simulink model "spring_mass_model_01"  (R2014a)
settings: Solver=FixedStepDiscrete  StartTime=0.0  StopTime=inf  FixedStep=sample_time  RelTol=1e-3
values from neighbouring files (symbols this model uses):
  g = g_real    (= 9.803)    [max_motor_torques.m]
  l0_leg = 0.97    [max_motor_torques.m]
  l0_virtual = sqrt(d^2+l0_leg^2-2*d*l0_leg*cos(phi0))    [max_motor_torques.m]
undefined symbols (not defined in the file or in its folder): alpha_apex, alpha_max, alpha_min, boom_mount_angle, c_energy, contact_threshold, control_start_time, d_y_boom_com_offset, d_y_boom_hip_offset, d_y_com, d_y_mount_to_com, desired_torso_angle, DiscIntNeverNeededParam, dt_thrust, dx_avg_desired, extra_leg_damping, F_thrust, fcut_contact, ff_energy_l, ff_energy_r, g_reduced, h_boom, i_limit_lateral, i_robot, initial_com_height, initial_dt, initial_dx, j_leg, j_rotor, j_segments, k0_virtual, k_placement, k_sea, kd_flight, kd_lateral, kd_leg_angle, kd_motor, kd_raibert, kd_torso, ki_lateral, kp_flight_max, kp_flight_min, kp_lateral, kp_leg_angle, kp_motor, kp_raibert, kp_torso, l0_max_angle_error, l0_min_angle_error, l0_min_flight_time, l_boom, l_boom_projected, l_max, l_min, l_retract_escape, l_retract_swing, l_seg, lambda1, lambda2, lateral_offset ... (+33)
libraries: simulink x22, simulink_extras x2
(part 1 of 3)
settings Model: xpc_rtwmakecfg_data=_xpcethercatlib_  BufferReuse=off  Creator=wmartin  LastModifiedBy=wmartin
settings SolverCC: EnableConcurrentExecution=on
settings DataIOCC: MaxDataPoints=1000000000  SaveFormat=StructureWithTime
settings OptimizationCC: BlockReduction=off  OptimizeBlockIOStorage=off  BufferReuse=off  GlobalBufferReuse=off  ExpressionFolding=off  ExpressionDepthLimit=2147483647  LocalBlockOutputs=off  SimCompilerOptimization=On
settings DebuggingCC: AlgebraicLoopMsg=error  UnderspecifiedInitializationDetection=Classic  StateNameClashWarn=warning
settings HardwareCC: ProdIntDivRoundTo=Zero  ProdEndianess=LittleEndian  ProdHWDeviceType=Generic->32-bit x86 compatible
settings ModelReferenceCC: UpdateModelReferenceTargets=IfOutOfDate  EnableParallelModelReferenceBuilds=on  ParallelModelReferenceMATLABWorkerInit=Copy Base Workspace
settings RTWCC: SystemTargetFile=slrt.tlc  TemplateMakefile=slrt_default_tmf  Description=Simulink Real-Time  RTWVerbose=off  ProcessScript=slrt_make_rtw_hook  RTWCompilerOptimization=On
settings CodeAppCC: MaxIdLength=127
settings TargetCC: CodeReplacementLibrary=XPC_BLAS  ParMdlRefBuildCompliant=on  ConcurrentExecutionCompliant=on  MatFileLogging=on  EnableShiftOperators=on  MATLABClassNameForMDSCustomization=xpcAperiodicCustomization

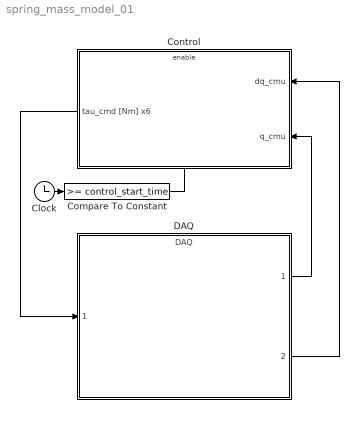
== system spring_mass_model_01 ==
  Clock : Clock
  Compare To Constant : simulink/Logic and Bit Operations/Compare To Constant  relop=>=  const=control_start_time  OutDataTypeStr=boolean
  Control : Subsystem
  DAQ : ModelReference  ModelNameDialog=DAQ  SimulationMode=Normal  ModelReferenceVersion=1.1655  CopyOfModelName=DAQ  DefaultDataLogging=on
  wires:
  DAQ/1 -> Control/2(q_cmu)
  DAQ/2 -> Control/1(dq_cmu)
  Clock/1 -> Compare To Constant/1
  Compare To Constant/1 -> Control/Enable
  Control/1(tau_cmd [Nm] x6) -> DAQ/1

== system spring_mass_model_01/Control ==
  dq_cmu : Inport
  q_cmu : Inport  Port=2
  Enable : EnablePort  StatesWhenEnabling=reset
  Actuator Control : ModelReference  ModelNameDialog=Actuator_Control  SimulationMode=Normal  ModelReferenceVersion=1.22  CopyOfModelName=Actuator_Control  DefaultDataLogging=on
  Behavior Control : Subsystem
  tau_cmd [Nm] x6 : Outport  InitialOutput=[0 0 0 0 0 0]
  wires:
  Behavior Control/1(Motor Torque Command [Nm] x6) -> Actuator Control/1
  dq_cmu/1 -> Behavior Control/1(dq_cmu), Actuator Control/4
  Actuator Control/1 -> tau_cmd [Nm] x6/1
  q_cmu/1 -> Behavior Control/2(q_cmu), Actuator Control/3
  Behavior Control/2(Force / Position Control [1/0] x4) -> Actuator Control/2

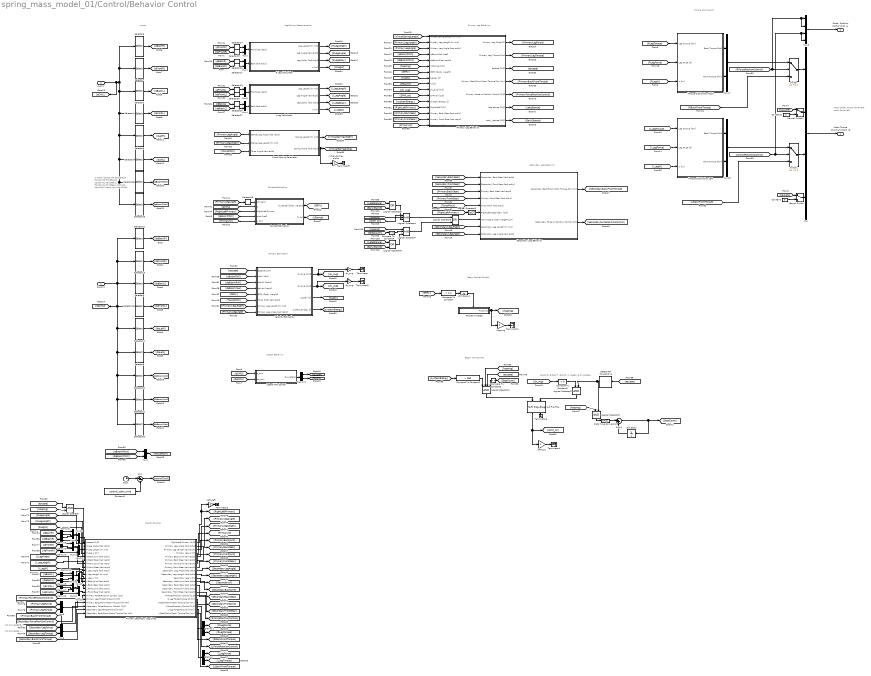
== system spring_mass_model_01/Control/Behavior Control ==
  note: not connected -->
  note: revert to raibert if velocity is negative on escape
  note: Motor Order:
      |
      | backR
      | frontR
      | latR
      | backL
      | frontL
      | latL
  note: q Order:
      |
      | backJointR
      | backGearR
      | frontJointR
      | frontGearR
      |
      | backJointL
      | backGearL
      | frontJointL
      | frontGearL
      |
      | latR
      | latL
      |
      | boomRoll
      | boomYaw
      | boomPitch
  note: Inputs
  note: Primary Leg Behavior
  note: Secondary Leg Behavior
  note: Torque Commands
  note: Lateral Behavior
  note: Leg/Spring Measurements
  note: Contact Estimation
  note: Velocity Estimation
  note: Begin SMM Control
  note: Begin Raibert Control
  note: Signal Routing
  note: not connected -->
  dq_cmu : Inport
  q_cmu : Inport  Port=2
  Clock : Clock
  Compare To Constant : simulink/Logic and Bit Operations/Compare To Constant  relop=>  const=1.4  OutDataTypeStr=boolean
  Compare To Constant1 : simulink/Logic and Bit Operations/Compare To Constant  relop=>  const=350  OutDataTypeStr=boolean
  Compare To Constant2 : simulink/Logic and Bit Operations/Compare To Constant  relop=<  const=0  OutDataTypeStr=boolean  ZeroCross=off
  Compare To Constant3 : simulink/Logic and Bit Operations/Compare To Constant  relop=>  const=4  OutDataTypeStr=boolean
  Compare To Constant4 : simulink/Logic and Bit Operations/Compare To Constant  relop=>  const=2  OutDataTypeStr=boolean
  Constant : Constant  Value=0
  Constant1 : Constant  Value=0
  Constant2 : Constant  Value=control_start_time
  Contact Estimation : Subsystem
  Data Type Conversion : DataTypeConversion  OutDataTypeStr=uint32
  Demux{,1..10} (11 alike) : Demux  Outputs=2
  Detect Fall Nonpositive : simulink/Logic and Bit Operations/Detect Fall Nonpositive  vinit=0  InputProcessing=Inherited  OutDataTypeStr=boolean
  L Leg Calculator : Subsystem
  Lateral PID Control : Subsystem
  Logical Operator : Logic  IconShape=distinctive  AllPortsSameDT=off  OutDataTypeStr=boolean
  Logical Operator1 : Logic  Inputs=4  IconShape=distinctive  AllPortsSameDT=off  OutDataTypeStr=boolean
  Logical Operator2 : Logic  IconShape=distinctive  AllPortsSameDT=off  OutDataTypeStr=boolean
  Logical Operator3 : Logic  Operator=NOT  AllPortsSameDT=off  OutDataTypeStr=boolean
  Logical Operator4 : Logic  Inputs=3  AllPortsSameDT=off  OutDataTypeStr=boolean
  Logical Operator5 : Logic  IconShape=distinctive  AllPortsSameDT=off  OutDataTypeStr=boolean
  Logical Operator6 : Logic  Operator=OR  AllPortsSameDT=off  OutDataTypeStr=boolean
  Logical Operator7 : Logic  Inputs=3  AllPortsSameDT=off  OutDataTypeStr=boolean
  Logical Operator8 : Logic  Operator=OR  AllPortsSameDT=off  OutDataTypeStr=boolean
  Logical Operator9 : Logic  Operator=OR  AllPortsSameDT=off  OutDataTypeStr=boolean
  Manual Switch : ManualSwitch
  Manual Switch1 : ManualSwitch
  Mux : Mux
  Mux{1..2,4..18} (17 alike) : Mux  Inputs=2
  Mux3 : Mux
  Primary Leg Behavior : Subsystem
  Primary Secondary Leg Swap : Subsystem
  R Leg Calculator : Subsystem
  Raibert Initiated : Subsystem
  S-R Flip-Flop : simulink_extras/Flip Flops/S-R Flip-Flop  initial_condition=0
  SMM_on : Gain
  Secondary Leg Behavior : Subsystem
  Selector1 : Selector  InputPortWidth=13  Indices=[10]
  Selector10 : Selector  InputPortWidth=13  Indices=[7 8]
  Selector11 : Selector  InputPortWidth=13  Indices=[9]
  Selector12 : Selector  InputPortWidth=13  Indices=[1 2]
  Selector13 : Selector  InputPortWidth=13  Indices=[3 4]
  Selector{14..17,19,24..27} (9 alike) : Selector  InputPortWidth=2  Indices=[1]
  Selector18 : Selector  InputPortWidth=13  Indices=[13]
  Selector2 : Selector  InputPortWidth=13  Indices=[5 6]
  Selector20 : Selector  InputPortWidth=13  Indices=[13]
  Selector21 : Selector  InputPortWidth=13  Indices=[11]
  Selector22 : Selector  InputPortWidth=13  Indices=[12]
  Selector23 : Selector  InputPortWidth=13  Indices=[11]
  Selector4 : Selector  InputPortWidth=13  Indices=[7 8]
  Selector5 : Selector  InputPortWidth=13  Indices=[9]
  Selector6 : Selector  InputPortWidth=13  Indices=[1 2]
  Selector7 : Selector  InputPortWidth=13  Indices=[3 4]
  Selector8 : Selector  InputPortWidth=13  Indices=[10]
  Selector9 : Selector  InputPortWidth=13  Indices=[5 6]
  Sum : Sum  Inputs=|+-
  Sum1 : Sum  Inputs=|++  OutMin=0
  Switch : Switch  Criteria=u2 ~= 0
  Switch1 : Switch  Criteria=u2 ~= 0
  Terminator{,1..6} (7 alike) : Terminator
  Torque Distribution Left : Subsystem
  Torque Distribution Right : Subsystem
  Unit Delay : UnitDelay  SampleTime=-1
  Unit Delay1 : UnitDelay  SampleTime=sample_time
  Velocity Estimation : Subsystem
  Virtual Spring Calculator : Subsystem
  dx_avg : Gain
  dy_avg : Gain
  hopping : Gain
  right_left : Gain
  virtual_spring_alpha : Gain
  Motor Torque Command [Nm] x6 : Outport  OutputWhenDisabled=reset  InitialOutput=[0 0 0 0 0 0]
  Force / Position Control [1/0] x4 : Outport  Port=2  OutputWhenDisabled=reset  InitialOutput=[0 0 0 0 0 0]
  wires:
  Lateral PID Control/1(tau_lateral) -> Demux2/1
  [dqCMU] -> Lateral PID Control/2(dq_cmu)
  [qCMU] -> Lateral PID Control/1(q_cmu)
  Sum/1 -> [controlClock]
  Selector4/1 -> [qFrontL]
  Selector2/1 -> [qBackL]
  Selector7/1 -> [qFrontR]
  Selector6/1 -> [qBackR]
  Selector1/1 -> [qLatL]
  Selector5/1 -> [qLatR]
  Constant2/1 -> Sum/2
  Clock/1 -> Sum/1
  Constant1/1 -> Manual Switch1/2
  Constant/1 -> Manual Switch/2
  Mux/1 -> Motor Torque Command [Nm] x6/1
  Selector8/1 -> [dqLatL]
  Selector11/1 -> [dqLatR]
  Selector12/1 -> [dqBackR]
  Selector13/1 -> [dqFrontR]
  Selector9/1 -> [dqBackL]
  Selector10/1 -> [dqFrontL]
  [qBackR] -> Selector16/1
  [dqBackR] -> Selector17/1
  [qFrontR] -> Selector14/1
  [dqFrontR] -> Selector15/1
  Mux2/1 -> R Leg Calculator/1(Front [rad rad/s])
  Mux1/1 -> R Leg Calculator/2(Back [rad rad/s])
  R Leg Calculator/1("Leg Length [m m/s] ") -> [RLegLength]
  R Leg Calculator/2(Leg Angle [rad rad/s]) -> [RLegAngle]
  R Leg Calculator/3(Leg Splay [rad rad/s]) -> [RLegSplay]
  Demux2/1 -> [tauLatR]
  Demux2/2 -> [tauLatL]
  [tauLatR] -> Manual Switch1/1
  [tauLatL] -> Manual Switch/1
  [RLegW] -> Torque Distribution Right/3(w [m])
  Selector14/1 -> Mux2/1
  Selector15/1 -> Mux2/2
  Selector17/1 -> Mux1/2
  Selector16/1 -> Mux1/1
  [PrimaryW] -> Contact Estimation/5(w [m])
  q_cmu/1 -> Selector6/1, Selector7/1, Selector2/1, Selector4/1, Selector5/1, Selector18/1, Selector23/1, Selector1/1, [qCMU]
  Selector18/1 -> [qBoomPitch]
  [qBoomPitch] -> Contact Estimation/4(pitch [rad])
  [PrimaryLegAngle] -> Selector19/1
  Selector19/1 -> Contact Estimation/1(phi [rad])
  Contact Estimation/1(F_vertical [body weight]) -> [GRFy]
  Selector20/1 -> [dqBoomPitch]
  [RLegForce] -> Torque Distribution Right/2(Leg Force [N])
  [RLegTorque] -> Torque Distribution Right/1(Leg Torque [Nm])
  Selector22/1 -> [dqBoomYaw]
  Contact Estimation/2(Ts [s]) -> [tStance]
  [GRFy] -> Compare To Constant/1
  Raibert Initiated/1(Hopping?) -> hopping/1, [hopping]
  dq_cmu/1 -> Selector20/1, Selector22/1, Selector21/1, Selector8/1, Selector11/1, Selector10/1, [dqCMU], Selector12/1, Selector13/1, Selector9/1
  Selector21/1 -> [dqBoomRoll]
  Selector23/1 -> [qBoomRoll]
  [qBackL] -> Selector26/1
  [dqBackL] -> Selector27/1
  [qFrontL] -> Selector24/1
  [dqFrontL] -> Selector25/1
  Mux5/1 -> L Leg Calculator/1(Front [rad rad/s])
  Mux4/1 -> L Leg Calculator/2(Back [rad rad/s])
  L Leg Calculator/1("Leg Length [m m/s] ") -> [LLegLength]
  L Leg Calculator/2(Leg Angle [rad rad/s]) -> [LLegAngle]
  L Leg Calculator/3(Leg Splay [rad rad/s]) -> [LLegSplay]
  Selector24/1 -> Mux5/1
  Selector25/1 -> Mux5/2
  Selector27/1 -> Mux4/2
  Selector26/1 -> Mux4/1
  R Leg Calculator/4(w [m]) -> [RLegW]
  L Leg Calculator/4(w [m]) -> [LLegW]
  Primary Leg Behavior/3(escape [1/0]) -> [escape]
  [PrimaryLegLength] -> Primary Leg Behavior/2(Primary Leg Length [m m/s])
  [hopping] -> Primary Leg Behavior/6(hopping [1/0])
  [GRFy] -> Primary Leg Behavior/7(GRFy [body weight])
  [qBoomPitch] -> Primary Leg Behavior/4(qBoomPitch [rad])
  [dqBoomPitch] -> Primary Leg Behavior/5(dqBoomPitch [rad/s])
  [PrimaryLegAngle] -> Primary Leg Behavior/3(Primary Leg Angle [rad rad/s])
  Primary Leg Behavior/1(Primary Leg Force [N]) -> [PrimaryLegForce]
  Primary Leg Behavior/2(Primary Leg Torque [Nm]) -> [PrimaryLegTorque]
  Velocity Estimation/1(dx_avg [m/s]) -> dx_avg/1, [dx_avg]
  [qBoomRoll] -> Velocity Estimation/2(qRoll [rad])
  [dqBoomYaw] -> Velocity Estimation/4(dqYaw [rad/s])
  dx_avg/1 -> Terminator/1
  hopping/1 -> Terminator1/1
  [LLegTorque] -> Torque Distribution Left/1(Leg Torque [Nm])
  [LLegForce] -> Torque Distribution Left/2(Leg Force [N])
  [LLegW] -> Torque Distribution Left/3(w [m])
  [qCMU] -> Contact Estimation/2(q)
  [RightLeftPrimary] -> Contact Estimation/3(Right/Left Primary)
  [PrimaryBackGear] -> Secondary Leg Behavior/3(Primary Back Gear [rad rad/s])
  [SecondaryLegAngle] -> Secondary Leg Behavior/9(Secondary Leg Angle [rad rad/s])
  [SecondaryLegLength] -> Secondary Leg Behavior/8(Secondary Leg Length [m m/s])
  right_left/1 -> Terminator2/1
  [hopping] -> Logical Operator/2
  Compare To Constant/1 -> Unit Delay1/1
  Velocity Estimation/2(dy_avg [m/s]) -> dy_avg/1, [dy_avg]
  [tApex] -> Primary Leg Behavior/8(t_apex [s])
  Velocity Estimation/3(t_apex [s]) -> [tApex]
  [GRFy] -> Velocity Estimation/5(GRFy [body weight])
  [PrimaryLegAngle] -> Velocity Estimation/8(Primary Leg Angle [rad rad/s])
  [PrimaryLegLength] -> Velocity Estimation/7(Primary Leg Length [m m/s])
  dy_avg/1 -> Terminator5/1
  [dqBoomRoll] -> Velocity Estimation/3(dqRoll [rad/s])
  [dx_avg] -> Primary Leg Behavior/10(dx_avg [m/s])
  [tStance] -> Primary Leg Behavior/9(Ts [s])
  Velocity Estimation/4(system_energy [J]) -> [systemEnergy]
  [systemEnergy] -> Compare To Constant1/1
  S-R Flip-Flop/1 -> [SMM_on], SMM_on/1
  SMM_on/1 -> Terminator4/1
  Compare To Constant1/1 -> Logical Operator1/1
  [SMM_on] -> Primary Leg Behavior/11(SMM On [1/0])
  [systemEnergy] -> Primary Leg Behavior/12(System Energy [J])
  Logical Operator1/1 -> S-R Flip-Flop/1
  [escape] -> Logical Operator1/3
  [RightLeftPrimary] -> Primary Leg Behavior/13(Right/Left [1/0])
  [PrimaryLegAngle] -> Virtual Spring Calculator/1("Stance Leg Angle [rad rad/s] ")
  [PrimaryLegLength] -> Virtual Spring Calculator/2(Stance Leg Length [m m/s])
  Virtual Spring Calculator/1(Spring Length [m m/s]) -> [VirtualSpringLength]
  [TorsoPitch] -> Virtual Spring Calculator/3(Torso Angle [rad rad/s])
  Virtual Spring Calculator/2(Spring Alpha [rad rad/s]) -> virtual_spring_alpha/1, [VirtualSpringAlpha]
  [qBoomPitch] -> Mux7/1
  [dqBoomPitch] -> Mux7/2
  Mux7/1 -> [TorsoPitch]
  [TorsoPitch] -> Secondary Leg Behavior/5(Torso Pitch [rad rad/s])
  [TorsoPitch] -> Velocity Estimation/6(Torso Pitch [rad rad/s])
  [VirtualSpringLength] -> Primary Leg Behavior/1(Virtual Spring Length [m m/s])
  virtual_spring_alpha/1 -> Terminator3/1
  [dx_avg] -> Compare To Constant2/1
  Detect Fall Nonpositive/1 -> Logical Operator2/2, Logical Operator5/2
  Compare To Constant2/1 -> Logical Operator2/1
  Logical Operator2/1 -> S-R Flip-Flop/2
  S-R Flip-Flop/2 -> Terminator6/1
  Mux3/1 -> Force / Position Control [1/0] x4/1
  Primary Secondary Leg Swap/2(Primary Leg Angle [rad rad/s]) -> [PrimaryLegAngle]
  Primary Secondary Leg Swap/4(Primary Leg w [m]) -> [PrimaryW]
  Primary Secondary Leg Swap/3(Primary Leg Length [rad rad/s]) -> [PrimaryLegLength]
  [RLegAngle] -> Primary Secondary Leg Swap/2(R Leg Angle [rad rad/s])
  [RLegLength] -> Primary Secondary Leg Swap/3(R Leg Length [m m/s])
  [RLegW] -> Primary Secondary Leg Swap/4(R Leg w [m])
  [LLegAngle] -> Primary Secondary Leg Swap/9(L Leg Angle [rad rad/s])
  [LLegLength] -> Primary Secondary Leg Swap/10(L Leg Length [m m/s])
  [LLegW] -> Primary Secondary Leg Swap/11(L Leg w [m])
  [SecondaryLegForce] -> Mux6/1
  [SecondaryLegTorque] -> Mux6/2
  Mux6/1 -> Primary Secondary Leg Swap/20(Secondary Leg Force/Torque [N Nm])
  Mux8/1 -> Primary Secondary Leg Swap/17(Primary Leg Force/Torque [N Nm])
  [PrimaryLegTorque] -> Mux8/2
  [PrimaryLegForce] -> Mux8/1
  Primary Secondary Leg Swap/10(Secondary Leg Length [rad rad/s]) -> [SecondaryLegLength]
  Primary Secondary Leg Swap/9(Secondary Leg Angle [rad rad/s]) -> [SecondaryLegAngle]
  Primary Secondary Leg Swap/20(L Leg Force/Torque [N Nm]) -> Demux/1
  Demux/1 -> [LLegForce]
  Demux/2 -> [LLegTorque]
  Primary Secondary Leg Swap/17(R Leg Force/Torque [N Nm]) -> Demux1/1
  Demux1/1 -> [RLegForce]
  Demux1/2 -> [RLegTorque]
  [qFrontR] -> Demux3/1
  [dqFrontR] -> Demux4/1
  Mux9/1 -> Primary Secondary Leg Swap/5(R Back Joint [rad rad/s])
  Mux10/1 -> Primary Secondary Leg Swap/6(R Back Gear [rad rad/s])
  Mux11/1 -> Primary Secondary Leg Swap/7(R Front Joint [rad rad/s])
  Mux12/1 -> Primary Secondary Leg Swap/8(R Front Gear [rad rad/s])
  Demux3/1 -> Mux11/1
  Demux3/2 -> Mux12/1
  Demux4/1 -> Mux11/2
  Demux4/2 -> Mux12/2
  [dqBackR] -> Demux5/1
  [qBackR] -> Demux6/1
  Demux6/1 -> Mux9/1
  Demux6/2 -> Mux10/1
  Demux5/1 -> Mux9/2
  Demux5/2 -> Mux10/2
  [qFrontL] -> Demux7/1
  [dqFrontL] -> Demux8/1
  Mux16/1 -> Primary Secondary Leg Swap/12(L Back Joint [rad rad/s])
  Mux13/1 -> Primary Secondary Leg Swap/13(L Back Gear [rad rad/s])
  Mux14/1 -> Primary Secondary Leg Swap/14(L Front Joint [rad rad/s])
  Mux15/1 -> Primary Secondary Leg Swap/15(L Front Gear [rad rad/s])
  Demux7/1 -> Mux14/1
  Demux7/2 -> Mux15/1
  Demux8/1 -> Mux14/2
  Demux8/2 -> Mux15/2
  [dqBackL] -> Demux9/1
  [qBackL] -> Demux10/1
  Demux10/1 -> Mux16/1
  Demux10/2 -> Mux13/1
  Demux9/1 -> Mux16/2
  Demux9/2 -> Mux13/2
  [PrimaryForcePositionControl] -> Primary Secondary Leg Swap/16(Primary Force/Position Control [1/0])
  [SecondaryForcePositionControl] -> Primary Secondary Leg Swap/19(Secondary Force/Position Control [1/0])
  [PrimaryBackFrontTorque] -> Primary Secondary Leg Swap/18(Primary Back/Front Motor Torque [Nm Nm])
  [SecondaryBackFrontTorque] -> Primary Secondary Leg Swap/21(Secondary Back/Front Motor Torque [Nm Nm])
  Primary Secondary Leg Swap/5(Primary Back Joint [rad rad/s]) -> [PrimaryBackJoint]
  Primary Secondary Leg Swap/6(Primary Back Gear [rad rad/s]) -> [PrimaryBackGear]
  Primary Secondary Leg Swap/7(Primary Front Joint [rad rad/s]) -> [PrimaryFrontJoint]
  Primary Secondary Leg Swap/8(Primary Front Gear [rad rad/s]) -> [PrimaryFrontGear]
  Primary Secondary Leg Swap/12(Secondary Back Joint [rad rad/s]) -> [SecondaryBackJoint]
  Primary Secondary Leg Swap/13(Secondary Back Gear [rad rad/s]) -> [SecondaryBackGear]
  Primary Secondary Leg Swap/14(Secondary Front Joint [rad rad/s]) -> [SecondaryFrontJoint]
  Primary Secondary Leg Swap/15(Secondary Front Gear [rad rad/s]) -> [SecondaryFrontGear]
  Primary Secondary Leg Swap/11(Secondary Leg w [m]) -> [SecondaryW]
  Primary Secondary Leg Swap/19(L Force/Position Control [1/0]) -> [LForcePositionControl]
  Primary Secondary Leg Swap/16(R Force/Position Control [1/0]) -> [RForcePositionControl]
  Primary Secondary Leg Swap/18(R Back/Front Motor Torque [Nm Nm]) -> [RBackFrontTorque]
  Primary Secondary Leg Swap/21(L Back/Front Motor Torque [Nm Nm]) -> [LBackFrontTorque]
  Logical Operator/1 -> Primary Secondary Leg Swap/1(escape [1/0])
  Primary Secondary Leg Swap/1(Right/Left Primary [1/0]) -> right_left/1, [RightLeftPrimary]
  [escape] -> Velocity Estimation/1(escape [1/0])
  [PrimaryBackGear] -> Primary Leg Behavior/14(Primary Back Gear [rad rad/s])
  [PrimaryFrontGear] -> Primary Leg Behavior/15(Primary Front Gear [rad rad/s])
  Primary Leg Behavior/4(Primary Back/Front Motor Torque [Nm Nm]) -> [PrimaryBackFrontTorque]
  Primary Leg Behavior/5(Primary Force or Position Control [1/0]) -> [PrimaryForcePositionControl]
  [PrimaryFrontGear] -> Secondary Leg Behavior/4(Primary Front Gear [rad rad/s])
  [RightLeftPrimary] -> Logical Operator3/1
  Logical Operator3/1 -> Secondary Leg Behavior/6(Right/Left Secondary [1/0])
  [SecondaryFrontGear] -> Secondary Leg Behavior/2(Secondary Front Gear [rad rad/s])
  [SecondaryBackGear] -> Secondary Leg Behavior/1(Secondary Back Gear [rad rad/s])
  Secondary Leg Behavior/2(Secondary Force or Position Control [1/0]) -> [SecondaryForcePositionControl]
  Secondary Leg Behavior/1(Secondary Back/Front Motor Torque [Nm Nm]) -> [SecondaryBackFrontTorque]
  Primary Leg Behavior/6(late stance [1/0]) -> [LateStance]
  [RForcePositionControl] -> Mux3/2, Mux3/1, Switch/2
  [LForcePositionControl] -> Mux3/4, Mux3/3, Switch1/2
  Switch/1 -> Mux/1
  Manual Switch1/1 -> Mux/2
  Manual Switch/1 -> Mux/4
  Torque Distribution Right/2(Front Torque [Nm]) -> Mux17/2
  Torque Distribution Right/1(Back Torque [Nm]) -> Mux17/1
  Torque Distribution Left/1(Back Torque [Nm]) -> Mux18/1
  Torque Distribution Left/2(Front Torque [Nm]) -> Mux18/2
  Mux17/1 -> Switch/1
  [RBackFrontTorque] -> Switch/3
  Mux18/1 -> Switch1/1
  [LBackFrontTorque] -> Switch1/3
  Switch1/1 -> Mux/3
  [PrimaryW] -> Primary Leg Behavior/16(Primary w [m])
  Logical Operator4/1 -> Logical Operator6/1
  [escape] -> Detect Fall Nonpositive/1
  [hopping] -> Logical Operator1/2
  Unit Delay/1 -> Sum1/2
  Sum1/1 -> [StepCount], Unit Delay/1
  Logical Operator5/1 -> Data Type Conversion/1
  Data Type Conversion/1 -> Sum1/1
  [hopping] -> Logical Operator5/1
  [StepCount] -> Compare To Constant3/1
  Compare To Constant3/1 -> Logical Operator1/4
  [StepCount] -> Compare To Constant4/1
  [hopping] -> Logical Operator7/1
  Compare To Constant4/1 -> Logical Operator7/2
  Logical Operator7/1 -> Logical Operator6/2
  Logical Operator6/1 -> Secondary Leg Behavior/7(Move Leg to Apex Target [1/0])
  Primary Leg Behavior/7(early_stance [1/0]) -> [EarlyStance]
  [EarlyStance] -> Logical Operator8/2
  [LateStance] -> Logical Operator8/1
  [EarlyStance] -> Logical Operator9/2
  [LateStance] -> Logical Operator9/1
  [hopping] -> Logical Operator4/1
  [SMM_on] -> Logical Operator4/2
  Logical Operator8/1 -> Logical Operator4/3
  Logical Operator9/1 -> Logical Operator7/3
  [escape] -> Logical Operator/1
  Unit Delay1/1 -> Raibert Initiated/Enable

== system spring_mass_model_01/Control/Behavior Control/Contact Estimation ==
  phi [rad] : Inport
  q : Inport  Port=2
  Right/Left Primary : Inport  Port=3
  pitch [rad] : Inport  Port=4
  w [m] : Inport  Port=5
  Compare To Constant : simulink/Logic and Bit Operations/Compare To Constant  relop=>=  const=loaded_threshold  OutDataTypeStr=boolean
  Compare To Constant1 : simulink/Logic and Bit Operations/Compare To Constant  relop=>=  const=0.040  OutDataTypeStr=boolean
  Constant : Constant  Value=m_total_real*g
  Contact Time : Subsystem
  Detect Decrease : simulink/Logic and Bit Operations/Detect Decrease  vinit=0.0  InputProcessing=Inherited  OutDataTypeStr=boolean
  Divide : Product  Inputs=*/
  Divide1 : Product  Inputs=*/
  Gain3 : Gain  Gain=-1
  Last Contact Time : Subsystem
  Leg Torque Measurements : Subsystem
  Logical Operator : Logic  AllPortsSameDT=off  OutDataTypeStr=boolean
  Sum1 : Sum  Inputs=|+-
  Vertical Spring Force : Subsystem
  two_pole_filter : DiscreteTransferFcn  Numerator=[(1-2*exp(-fcut_contact*sample_time)+exp(-2*fcut_contact*sample_time)) 0 0]  Denominator=[1 (-2*exp(-fcut_contact*sample_time)) (exp(-2*fcut_contact*sample_time))]  SampleTime=sample_time
  F_vertical [body weight] : Outport
  Ts [s] : Outport  Port=2
  wires:
  Vertical Spring Force/1(Vertical Force [N]) -> two_pole_filter/1
  Constant/1 -> Divide/2
  two_pole_filter/1 -> Divide/1
  q/1 -> Leg Torque Measurements/1(q)
  Leg Torque Measurements/1(Back [Nm]) -> Sum1/1
  Leg Torque Measurements/2(Front [Nm]) -> Sum1/2
  Sum1/1 -> Divide1/1
  Divide1/1 -> Vertical Spring Force/3(Force [N])
  pitch [rad]/1 -> Vertical Spring Force/1(theta [rad])
  w [m]/1 -> Gain3/1
  Gain3/1 -> Divide1/2
  phi [rad]/1 -> Vertical Spring Force/2(phi [rad])
  Last Contact Time/1(Ts [s]) -> Ts [s]/1
  Contact Time/1(ts [s]) -> Last Contact Time/1(ts [s]), Compare To Constant1/1
  Compare To Constant/1 -> Detect Decrease/1, Contact Time/Enable
  Logical Operator/1 -> Last Contact Time/Trigger
  Detect Decrease/1 -> Logical Operator/1
  Compare To Constant1/1 -> Logical Operator/2
  Right/Left Primary/1 -> Leg Torque Measurements/2(Right/Left Stance [1/0])
  Divide/1 -> F_vertical [body weight]/1, Compare To Constant/1

== system spring_mass_model_01/Control/Behavior Control/L Leg Calculator ==
  Front [rad rad/s] : Inport
  Back [rad rad/s] : Inport  Port=2
  Demux1 : Demux  Outputs=2
  Gain1 : Gain  Gain=2*l_seg
  Gain2 : Gain  Gain=l_seg
  Gain3 : Gain  Gain=-1
  Gain4 : Gain  Gain=0.5
  Gain5 : Gain  Gain=0.5
  Gain6 : Gain  Gain=2
  Mux1 : Mux  Inputs=2
  Product : Product  RndMeth=Zero
  Sum4 : Sum  Inputs=+|+
  Sum5 : Sum  Inputs=+|-
  Trigonometric Function : Trigonometry  Operator=cos
  Trigonometric Function1 : Trigonometry
  "Leg Length [m m/s] " : Outport
  Leg Angle [rad rad/s] : Outport  Port=2
  Leg Splay [rad rad/s] : Outport  Port=3
  w [m] : Outport  Port=4
  wires:
  Gain5/1 -> Leg Angle [rad rad/s]/1
  Sum4/1 -> Gain5/1
  Mux1/1 -> "Leg Length [m m/s] "/1
  Sum5/1 -> Demux1/1, Leg Splay [rad rad/s]/1
  Gain2/1 -> Gain6/1, Product/1
  Demux1/1 -> Gain4/1
  Gain3/1 -> Product/2
  Demux1/2 -> Gain3/1
  Back [rad rad/s]/1 -> Sum5/1, Sum4/1
  Front [rad rad/s]/1 -> Sum4/2, Sum5/2
  Product/1 -> Mux1/2
  Trigonometric Function1/1 -> Gain2/1
  Gain1/1 -> Mux1/1
  Trigonometric Function/1 -> Gain1/1
  Gain4/1 -> Trigonometric Function/1, Trigonometric Function1/1
  Gain6/1 -> w [m]/1

== system spring_mass_model_01/Control/Behavior Control/Lateral PID Control ==
  note: FB Linearization
  q_cmu : Inport
  dq_cmu : Inport  Port=2
  -mgd : Gain  Gain=m_leg_motor*g*lateral_offset
  90deg : Constant  Value=pi/2
  Gain : Gain  Gain=-1
  Lateral Hip PID : Subsystem
  Motor Saturation : Saturate  UpperLimit=max_torque_lateral  LowerLimit=-max_torque_lateral
      settings: AttributesFormatString=Top: %<UpperLimit>\nBottom: %<LowerLimit>
  Mux : Mux  Inputs=2
  Sum1 : Sum  Inputs=|+-
  Sum2 : Sum  Inputs=-+|
  Sum3 : Sum  Inputs=++|
  Sum4 : Sum  Inputs=++|
  desired_velocity : Constant  Value=0
  lateral_sine : Gain  Commented=on  Gain=pi/180
  lateral_wave : Sin  Commented=on  Amplitude=5  Frequency=2*pi*(1/2)  SampleTime=0
  select_dqLateral : Selector  InputPortWidth=13  Indices=[9 10]
  select_qLateral : Selector  InputPortWidth=13  Indices=[9 10]
  sin : Trigonometry
  spherical_correction_angle : Subsystem
  tau_lateral : Outport
  wires:
  lateral_wave/1 -> lateral_sine/1
  Lateral Hip PID/1(out) -> Sum4/2
  Sum2/1 -> Lateral Hip PID/1(position_error)
  q_cmu/1 -> spherical_correction_angle/1(q_cmu), select_qLateral/1
  select_dqLateral/1 -> Sum1/2
  dq_cmu/1 -> select_dqLateral/1
  Sum4/1 -> Motor Saturation/1
  desired_velocity/1 -> Sum1/1
  Sum1/1 -> Lateral Hip PID/2(velocity_error)
  Gain/1 -> Mux/2
  Mux/1 -> Sum2/2
  select_qLateral/1 -> Sum3/2, Sum2/1  "qLateral"
  Motor Saturation/1 -> tau_lateral/1
  spherical_correction_angle/1(lateral_correction [rad]) -> Mux/1, Gain/1
  -mgd/1 -> Sum4/1
  Sum3/1 -> sin/1
  90deg/1 -> Sum3/1
  sin/1 -> -mgd/1

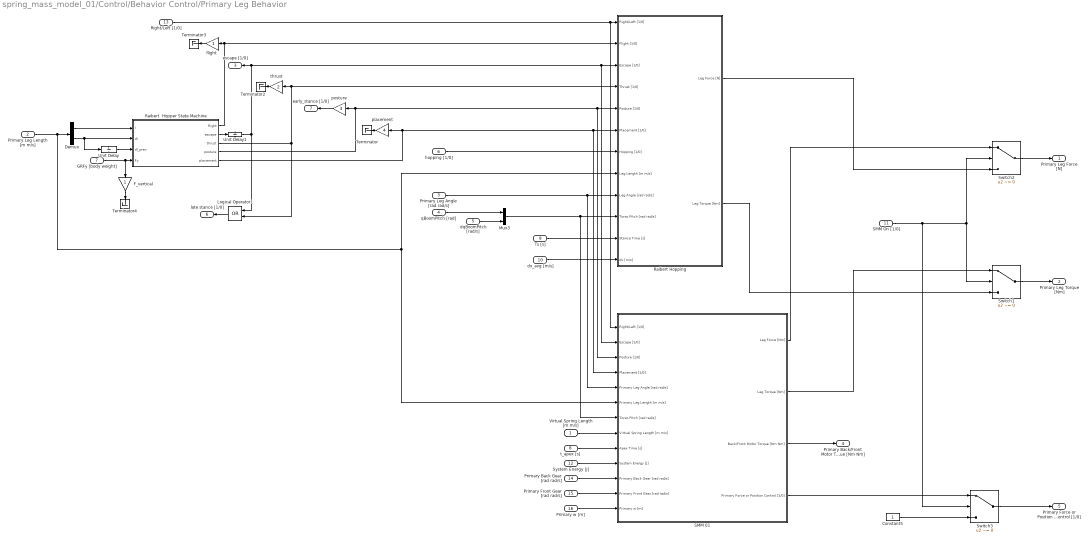
== system spring_mass_model_01/Control/Behavior Control/Primary Leg Behavior ==
  Virtual Spring Length [m m/s] : Inport
  Primary Leg Length [m m/s] : Inport  Port=2
  Primary Leg Angle [rad rad/s] : Inport  Port=3
  qBoomPitch [rad] : Inport  Port=4
  dqBoomPitch [rad/s] : Inport  Port=5
  hopping [1/0] : Inport  Port=6
  GRFy [body weight] : Inport  Port=7
  t_apex [s] : Inport  Port=8
  Ts [s] : Inport  Port=9
  dx_avg [m/s] : Inport  Port=10
  SMM On [1/0] : Inport  Port=11
  System Energy [J] : Inport  Port=12
  Right/Left [1/0] : Inport  Port=13
  Primary Back Gear [rad rad/s] : Inport  Port=14
  Primary Front Gear [rad rad/s] : Inport  Port=15
  Primary w [m] : Inport  Port=16
  Constant5 : Constant  OutDataTypeStr=boolean
  Demux : Demux  Outputs=2
  F_vertical : Gain
  Logical Operator1 : Logic  Operator=OR  AllPortsSameDT=off  OutDataTypeStr=boolean
  Mux3 : Mux  Inputs=2
  Raibert  Hopper State Machine : State Transition Table  TreatAsAtomicUnit=on
  Raibert Hopping : Subsystem
  SMM 01 : Subsystem
  Switch1 : Switch  Criteria=u2 ~= 0
  Switch2 : Switch  Criteria=u2 ~= 0
  Switch3 : Switch  Criteria=u2 ~= 0
  Terminator{,2..4} (4 alike) : Terminator
  Unit Delay : UnitDelay  SampleTime=-1
  Unit Delay1 : UnitDelay  SampleTime=sample_time
  flight : Gain
  placement : Gain  Gain=4
  posture : Gain  Gain=3
  thrust : Gain  Gain=2
  Primary Leg Force [N] : Outport
  Primary Leg Torque [Nm] : Outport  Port=2
  escape [1/0] : Outport  Port=3
  Primary Back/Front Motor Torque [Nm Nm] : Outport  Port=4
  Primary Force or Position Control [1/0] : Outport  Port=5
  late stance [1/0] : Outport  Port=6
  early_stance [1/0] : Outport  Port=7
  wires:
  Raibert  Hopper State Machine/4(posture) -> posture/1, SMM 01/3(Posture [1/0]), Raibert Hopping/5(Posture [1/0])
  Mux3/1 -> SMM 01/7(Torso Pitch [rad rad/s]), Raibert Hopping/10(Torso Pitch [rad rad/s])
  qBoomPitch [rad]/1 -> Mux3/1
  dqBoomPitch [rad/s]/1 -> Mux3/2
  Unit Delay/1 -> Raibert  Hopper State Machine/3(dl_prev)
  GRFy [body weight]/1 -> F_vertical/1, Raibert  Hopper State Machine/4(Fy)
  Demux/2 -> Unit Delay/1, Raibert  Hopper State Machine/2(dl)
  Raibert  Hopper State Machine/3(thrust) -> Logical Operator1/2, Raibert Hopping/4(Thrust [1/0]), thrust/1
  Raibert  Hopper State Machine/1(flight) -> flight/1, Raibert Hopping/2(Flight [1/0])
  Raibert  Hopper State Machine/5(placement) -> Raibert Hopping/6(Placement [1/0]), SMM 01/4(Placement [1/0]), placement/1
  placement/1 -> Terminator/1
  posture/1 -> early_stance [1/0]/1
  thrust/1 -> Terminator2/1
  Primary Leg Length [m m/s]/1 -> SMM 01/6(Primary Leg Length [m m/s]), Raibert Hopping/8(Leg Length [m m/s]), Demux/1
  F_vertical/1 -> Terminator4/1
  flight/1 -> Terminator3/1
  Demux/1 -> Raibert  Hopper State Machine/1(l)
  hopping [1/0]/1 -> Raibert Hopping/7(Hopping [1/0])
  SMM On [1/0]/1 -> Switch3/2, Switch1/2, Switch2/2
  Ts [s]/1 -> Raibert Hopping/11(Stance Time [s])
  dx_avg [m/s]/1 -> Raibert Hopping/12(dx [m/s])
  Raibert Hopping/1(Leg Force [N]) -> Switch2/3
  Raibert Hopping/2(Leg Torque [Nm]) -> Switch1/3
  Switch2/1 -> Primary Leg Force [N]/1
  Switch1/1 -> Primary Leg Torque [Nm]/1
  t_apex [s]/1 -> SMM 01/9(Apex Time [s])
  System Energy [J]/1 -> SMM 01/10(System Energy [J])
  SMM 01/1(Leg Force [Nm]) -> Switch2/1
  SMM 01/2(Leg Torque [Nm]) -> Switch1/1
  Right/Left [1/0]/1 -> SMM 01/1(Right/Left [1/0]), Raibert Hopping/1(Right/Left [1/0])
  Virtual Spring Length [m m/s]/1 -> SMM 01/8(Virtual Spring Length [m m/s])
  Primary Front Gear [rad rad/s]/1 -> SMM 01/12(Primary Front Gear [rad rad/s])
  Primary Back Gear [rad rad/s]/1 -> SMM 01/11(Primary Back Gear [rad rad/s])
  Primary Leg Angle [rad rad/s]/1 -> SMM 01/5(Primary Leg Angle [rad rad/s]), Raibert Hopping/9(Leg Angle [rad rad/s])
  SMM 01/3(Back/Front Motor Torque [Nm Nm]) -> Primary Back/Front Motor Torque [Nm Nm]/1
  Logical Operator1/1 -> late stance [1/0]/1
  Switch3/1 -> Primary Force or Position Control [1/0]/1
  Constant5/1 -> Switch3/3
  SMM 01/4(Primary Force or Position Control [1/0]) -> Switch3/1
  Primary w [m]/1 -> SMM 01/13(Primary w [m])
  Raibert  Hopper State Machine/2(escape) -> Unit Delay1/1
  Unit Delay1/1 -> SMM 01/2(Escape [1/0]), Raibert Hopping/3(Escape [1/0]), escape [1/0]/1, Logical Operator1/1

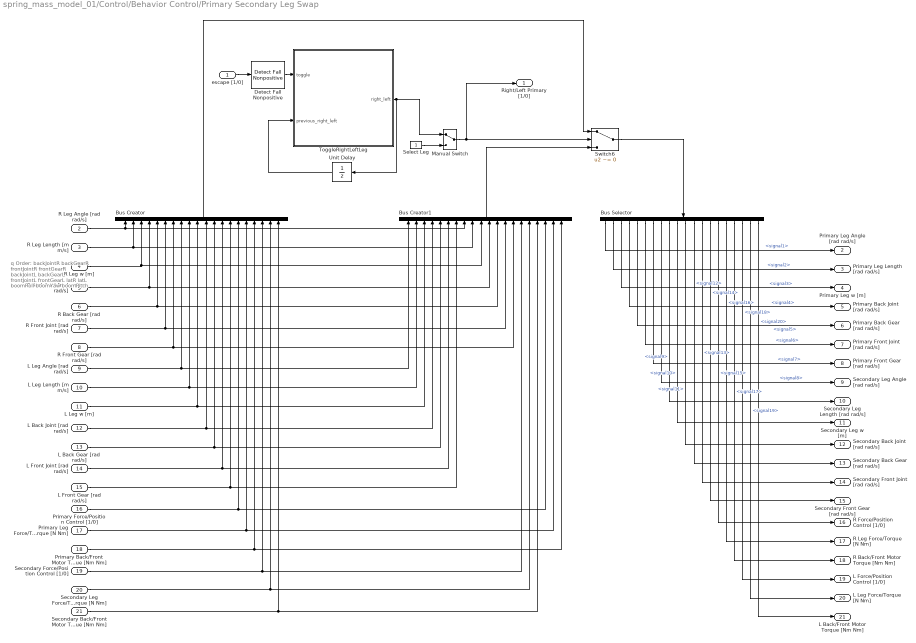
== system spring_mass_model_01/Control/Behavior Control/Primary Secondary Leg Swap ==
  note: q Order:
      |
      | backJointR
      | backGearR
      | frontJointR
      | frontGearR
      |
      | backJointL
      | backGearL
      | frontJointL
      | frontGearL
      |
      | latR
      | latL
      |
      | boomRoll
      | boomYaw
      | boomPitch
  escape [1/0] : Inport
  R Leg Angle [rad rad/s] : Inport  Port=2
  R Leg Length [m m/s] : Inport  Port=3
  R Leg w [m] : Inport  Port=4
  R Back Joint [rad rad/s] : Inport  Port=5
  R Back Gear [rad rad/s] : Inport  Port=6
  R Front Joint [rad rad/s] : Inport  Port=7
  R Front Gear [rad rad/s] : Inport  Port=8
  L Leg Angle [rad rad/s] : Inport  Port=9
  L Leg Length [m m/s] : Inport  Port=10
  L Leg w [m] : Inport  Port=11
  L Back Joint [rad rad/s] : Inport  Port=12
  L Back Gear [rad rad/s] : Inport  Port=13
  L Front Joint [rad rad/s] : Inport  Port=14
  L Front Gear [rad rad/s] : Inport  Port=15
  Primary Force/Position Control [1/0] : Inport  Port=16
  Primary Leg Force/Torque [N Nm] : Inport  Port=17
  Primary Back/Front Motor Torque [Nm Nm] : Inport  Port=18
  Secondary Force/Position Control [1/0] : Inport  Port=19
  Secondary Leg Force/Torque [N Nm] : Inport  Port=20
  Secondary Back/Front Motor Torque [Nm Nm] : Inport  Port=21
  Bus Creator : BusCreator  Inputs=20
  Bus Creator1 : BusCreator  Inputs=20
  Bus Selector : BusSelector  OutputSignals=signal1,signal2,signal3,signal4,signal5,signal6,signal7,signal8,signal9,signal10,signal11,signal12,signal13,signal14,signal15,signal16,signal17,signal18,signal19,signal20
  Detect Fall Nonpositive : simulink/Logic and Bit Operations/Detect Fall Nonpositive  vinit=0  InputProcessing=Inherited  OutDataTypeStr=boolean
  Manual Switch : ManualSwitch
  Select Leg : Constant  OutDataTypeStr=boolean
  Switch6 : Switch  Criteria=u2 ~= 0  OutDataTypeStr=Inherit: Inherit via back propagation  ZeroCross=off
  ToggleRightLeftLeg : MATLAB Function  TreatAsAtomicUnit=on
      settings: MinAlgLoopOccurrences=on
  Unit Delay : UnitDelay  SampleTime=sample_time
  Right/Left Primary [1/0] : Outport
  Primary Leg Angle [rad rad/s] : Outport  Port=2
  Primary Leg Length [rad rad/s] : Outport  Port=3
  Primary Leg w [m] : Outport  Port=4
  Primary Back Joint [rad rad/s] : Outport  Port=5
  Primary Back Gear [rad rad/s] : Outport  Port=6
  Primary Front Joint [rad rad/s] : Outport  Port=7
  Primary Front Gear [rad rad/s] : Outport  Port=8
  Secondary Leg Angle [rad rad/s] : Outport  Port=9
  Secondary Leg Length [rad rad/s] : Outport  Port=10
  Secondary Leg w [m] : Outport  Port=11
  Secondary Back Joint [rad rad/s] : Outport  Port=12
  Secondary Back Gear [rad rad/s] : Outport  Port=13
  Secondary Front Joint [rad rad/s] : Outport  Port=14
  Secondary Front Gear [rad rad/s] : Outport  Port=15
  R Force/Position Control [1/0] : Outport  Port=16
  R Leg Force/Torque [N Nm] : Outport  Port=17
  R Back/Front Motor Torque [Nm Nm] : Outport  Port=18
  L Force/Position Control [1/0] : Outport  Port=19
  L Leg Force/Torque [N Nm] : Outport  Port=20
  L Back/Front Motor Torque [Nm Nm] : Outport  Port=21
  wires:
  Bus Selector/20 -> L Back/Front Motor Torque [Nm Nm]/1  "<signal20>"
  Bus Selector/19 -> L Leg Force/Torque [N Nm]/1  "<signal19>"
  Bus Selector/18 -> L Force/Position Control [1/0]/1  "<signal18>"
  Bus Selector/17 -> R Back/Front Motor Torque [Nm Nm]/1  "<signal17>"
  Bus Selector/16 -> R Leg Force/Torque [N Nm]/1  "<signal16>"
  Bus Selector/15 -> R Force/Position Control [1/0]/1  "<signal15>"
  Bus Selector/14 -> Secondary Front Gear [rad rad/s]/1  "<signal14>"
  Bus Selector/13 -> Secondary Front Joint [rad rad/s]/1  "<signal13>"
  Bus Selector/12 -> Secondary Back Gear [rad rad/s]/1  "<signal12>"
  Bus Selector/11 -> Secondary Back Joint [rad rad/s]/1  "<signal11>"
  Bus Selector/10 -> Secondary Leg w [m]/1  "<signal10>"
  Bus Selector/9 -> Secondary Leg Length [rad rad/s]/1  "<signal9>"
  Bus Selector/8 -> Secondary Leg Angle [rad rad/s]/1  "<signal8>"
  Bus Selector/7 -> Primary Front Gear [rad rad/s]/1  "<signal7>"
  Bus Selector/6 -> Primary Front Joint [rad rad/s]/1  "<signal6>"
  Bus Selector/5 -> Primary Back Gear [rad rad/s]/1  "<signal5>"
  Bus Selector/4 -> Primary Back Joint [rad rad/s]/1  "<signal4>"
  Bus Selector/3 -> Primary Leg w [m]/1  "<signal3>"
  Bus Selector/2 -> Primary Leg Length [rad rad/s]/1  "<signal2>"
  Bus Selector/1 -> Primary Leg Angle [rad rad/s]/1  "<signal1>"
  Switch6/1 -> Bus Selector/1
  Secondary Back/Front Motor Torque [Nm Nm]/1 -> Bus Creator/20, Bus Creator1/17
  Secondary Leg Force/Torque [N Nm]/1 -> Bus Creator/19, Bus Creator1/16
  Secondary Force/Position Control [1/0]/1 -> Bus Creator/18, Bus Creator1/15
  Primary Back/Front Motor Torque [Nm Nm]/1 -> Bus Creator/17, Bus Creator1/20
  Primary Leg Force/Torque [N Nm]/1 -> Bus Creator/16, Bus Creator1/19
  Primary Force/Position Control [1/0]/1 -> Bus Creator/15, Bus Creator1/18
  L Front Gear [rad rad/s]/1 -> Bus Creator/14, Bus Creator1/7
  L Front Joint [rad rad/s]/1 -> Bus Creator1/6, Bus Creator/13
  L Back Gear [rad rad/s]/1 -> Bus Creator/12, Bus Creator1/5
  L Back Joint [rad rad/s]/1 -> Bus Creator/11, Bus Creator1/4
  L Leg w [m]/1 -> Bus Creator/10, Bus Creator1/3
  L Leg Length [m m/s]/1 -> Bus Creator/9, Bus Creator1/2
  L Leg Angle [rad rad/s]/1 -> Bus Creator/8, Bus Creator1/1
  R Front Gear [rad rad/s]/1 -> Bus Creator/7, Bus Creator1/14
  R Front Joint [rad rad/s]/1 -> Bus Creator/6, Bus Creator1/13
  R Back Gear [rad rad/s]/1 -> Bus Creator/5, Bus Creator1/12
  R Back Joint [rad rad/s]/1 -> Bus Creator/4, Bus Creator1/11
  Bus Creator1/1 -> Switch6/3
  Bus Creator/1 -> Switch6/1
  R Leg Length [m m/s]/1 -> Bus Creator/2, Bus Creator1/9
  R Leg Angle [rad rad/s]/1 -> Bus Creator/1, Bus Creator1/8
  R Leg w [m]/1 -> Bus Creator/3, Bus Creator1/10
  Select Leg/1 -> Manual Switch/2
  Manual Switch/1 -> Switch6/2, Right/Left Primary [1/0]/1
  ToggleRightLeftLeg/1(right_left) -> Manual Switch/1, Unit Delay/1
  escape [1/0]/1 -> Detect Fall Nonpositive/1
  Detect Fall Nonpositive/1 -> ToggleRightLeftLeg/1(toggle)
  Unit Delay/1 -> ToggleRightLeftLeg/2(previous_right_left)

== system spring_mass_model_01/Control/Behavior Control/R Leg Calculator ==
  Front [rad rad/s] : Inport
  Back [rad rad/s] : Inport  Port=2
  Demux1 : Demux  Outputs=2
  Gain1 : Gain  Gain=2*l_seg
  Gain2 : Gain  Gain=l_seg
  Gain3 : Gain  Gain=-1
  Gain4 : Gain  Gain=0.5
  Gain5 : Gain  Gain=0.5
  Gain6 : Gain  Gain=2
  Mux1 : Mux  Inputs=2
  Product : Product  RndMeth=Zero
  Sum4 : Sum  Inputs=+|+
  Sum5 : Sum  Inputs=+|-
  Trigonometric Function : Trigonometry  Operator=cos
  Trigonometric Function1 : Trigonometry
  "Leg Length [m m/s] " : Outport
  Leg Angle [rad rad/s] : Outport  Port=2
  Leg Splay [rad rad/s] : Outport  Port=3
  w [m] : Outport  Port=4
  wires:
  Gain6/1 -> w [m]/1
  Gain4/1 -> Trigonometric Function1/1, Trigonometric Function/1
  Trigonometric Function/1 -> Gain1/1
  Gain1/1 -> Mux1/1
  Trigonometric Function1/1 -> Gain2/1
  Product/1 -> Mux1/2
  Front [rad rad/s]/1 -> Sum5/2, Sum4/2
  Back [rad rad/s]/1 -> Sum4/1, Sum5/1
  Demux1/2 -> Gain3/1
  Gain3/1 -> Product/2
  Demux1/1 -> Gain4/1
  Gain2/1 -> Product/1, Gain6/1
  Sum5/1 -> Leg Splay [rad rad/s]/1, Demux1/1
  Mux1/1 -> "Leg Length [m m/s] "/1
  Sum4/1 -> Gain5/1
  Gain5/1 -> Leg Angle [rad rad/s]/1

== system spring_mass_model_01/Control/Behavior Control/Raibert Initiated ==
  Enable : EnablePort  StatesWhenEnabling=reset
  Constant : Constant
  Hopping? : Outport  InitialOutput=[0]
  wires:
  Constant/1 -> Hopping?/1

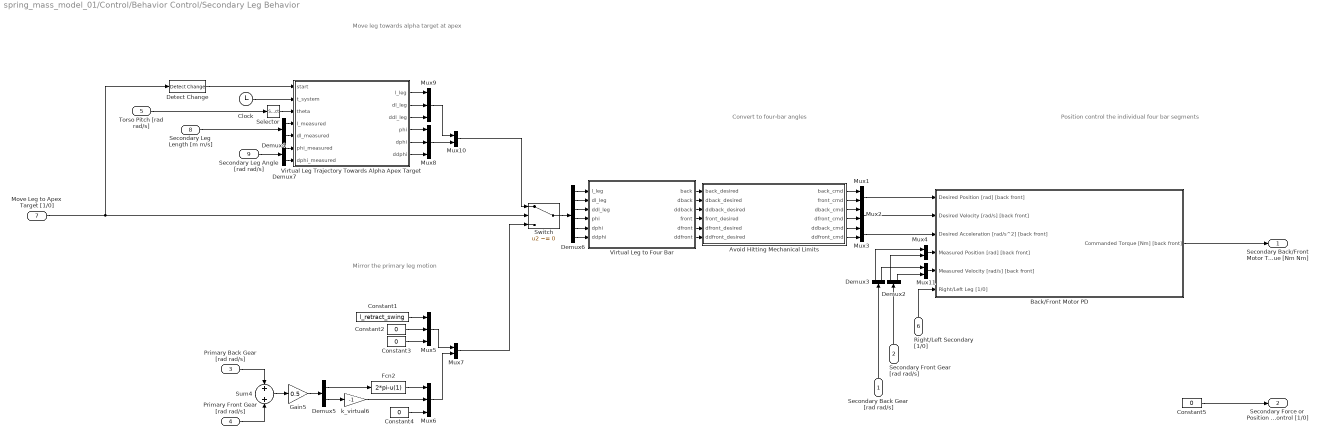
== system spring_mass_model_01/Control/Behavior Control/Secondary Leg Behavior ==
  note: Convert to
      | four-bar angles
  note: Position control the
      | individual four bar segments
  note: Move leg towards
      | alpha target at apex
  note: Mirror the primary
      | leg motion
  Secondary Back Gear [rad rad/s] : Inport
  Secondary Front Gear [rad rad/s] : Inport  Port=2
  Primary Back Gear [rad rad/s] : Inport  Port=3
  Primary Front Gear [rad rad/s] : Inport  Port=4
  Torso Pitch [rad rad/s] : Inport  Port=5
  Right/Left Secondary [1/0] : Inport  Port=6
  Move Leg to Apex Target [1/0] : Inport  Port=7
  Secondary Leg Length [m m/s] : Inport  Port=8
  Secondary Leg Angle [rad rad/s] : Inport  Port=9
  Avoid Hitting Mechanical Limits : MATLAB Function  TreatAsAtomicUnit=on
  Back/Front Motor PD : Subsystem
  Clock : Clock
  Constant1 : Constant  Value=l_retract_swing
  Constant2 : Constant  Value=0
  Constant3 : Constant  Value=0
  Constant4 : Constant  Value=0
  Constant5 : Constant  Value=0  OutDataTypeStr=boolean
  Demux{2..5,7} (5 alike) : Demux  Outputs=2
  Demux6 : Demux  Outputs=6
  Detect Change : simulink/Logic and Bit Operations/Detect Change  vinit=0  InputProcessing=Inherited  OutDataTypeStr=boolean
  Fcn2 : Fcn  Expr=2*pi-u(1)
  Gain5 : Gain  Gain=0.5
  Mux{1..4,7,10..11} (7 alike) : Mux  Inputs=2
  Mux{5..6,8..9} (4 alike) : Mux  Inputs=3
  Selector : Selector  InputPortWidth=2  Indices=[1]
  Sum4 : Sum  Inputs=+|+
  Switch : Switch  Criteria=u2 ~= 0
  Virtual Leg Trajectory Towards Alpha Apex Target : MATLAB Function  TreatAsAtomicUnit=on
  Virtual Leg to Four Bar : MATLAB Function  TreatAsAtomicUnit=on
  k_virtual6 : Gain  Gain=-1
  Secondary Back/Front Motor Torque [Nm Nm] : Outport
  Secondary Force or Position Control [1/0] : Outport  Port=2
  wires:
  Mux3/1 -> Back/Front Motor PD/3(Desired Acceleration [rad/s^2] [back front])
  Mux2/1 -> Back/Front Motor PD/2(Desired Velocity [rad/s] [back front])
  Avoid Hitting Mechanical Limits/6(ddfront_cmd) -> Mux3/2
  Avoid Hitting Mechanical Limits/5(ddback_cmd) -> Mux3/1
  Avoid Hitting Mechanical Limits/4(dfront_cmd) -> Mux2/2
  Avoid Hitting Mechanical Limits/3(dback_cmd) -> Mux2/1
  Secondary Back Gear [rad rad/s]/1 -> Demux3/1
  Secondary Front Gear [rad rad/s]/1 -> Demux2/1
  Demux2/1 -> Mux4/2
  Avoid Hitting Mechanical Limits/1(back_cmd) -> Mux1/1
  Avoid Hitting Mechanical Limits/2(front_cmd) -> Mux1/2
  Demux3/1 -> Mux4/1
  Demux3/2 -> Mux11/1
  Right/Left Secondary [1/0]/1 -> Back/Front Motor PD/6(Right/Left Leg [1/0])
  Mux1/1 -> Back/Front Motor PD/1(Desired Position [rad] [back front])
  Mux4/1 -> Back/Front Motor PD/4(Measured Position [rad] [back front])
  Demux2/2 -> Mux11/2
  Mux11/1 -> Back/Front Motor PD/5(Measured Velocity [rad/s] [back front])
  Demux6/6 -> Virtual Leg to Four Bar/6(ddphi)
  Demux6/5 -> Virtual Leg to Four Bar/5(dphi)
  Demux6/4 -> Virtual Leg to Four Bar/4(phi)
  Demux6/3 -> Virtual Leg to Four Bar/3(ddl_leg)
  Demux6/2 -> Virtual Leg to Four Bar/2(dl_leg)
  Demux6/1 -> Virtual Leg to Four Bar/1(l_leg)
  Virtual Leg to Four Bar/6(ddfront) -> Avoid Hitting Mechanical Limits/6(ddfront_desired)
  Virtual Leg to Four Bar/5(dfront) -> Avoid Hitting Mechanical Limits/5(dfront_desired)
  Virtual Leg to Four Bar/4(front) -> Avoid Hitting Mechanical Limits/4(front_desired)
  Virtual Leg to Four Bar/3(ddback) -> Avoid Hitting Mechanical Limits/3(ddback_desired)
  Virtual Leg to Four Bar/2(dback) -> Avoid Hitting Mechanical Limits/2(dback_desired)
  Virtual Leg to Four Bar/1(back) -> Avoid Hitting Mechanical Limits/1(back_desired)
  Secondary Leg Angle [rad rad/s]/1 -> Demux7/1
  Secondary Leg Length [m m/s]/1 -> Demux4/1
  Demux7/2 -> Virtual Leg Trajectory Towards Alpha Apex Target/7(dphi_measured)
  Demux7/1 -> Virtual Leg Trajectory Towards Alpha Apex Target/6(phi_measured)
  Demux4/1 -> Virtual Leg Trajectory Towards Alpha Apex Target/4(l_measured)
  Demux4/2 -> Virtual Leg Trajectory Towards Alpha Apex Target/5(dl_measured)
  Clock/1 -> Virtual Leg Trajectory Towards Alpha Apex Target/2(t_system)
  Detect Change/1 -> Virtual Leg Trajectory Towards Alpha Apex Target/1(start)
  Virtual Leg Trajectory Towards Alpha Apex Target/1(l_leg) -> Mux9/1
  Virtual Leg Trajectory Towards Alpha Apex Target/2(dl_leg) -> Mux9/2
  Virtual Leg Trajectory Towards Alpha Apex Target/3(ddl_leg) -> Mux9/3
  Virtual Leg Trajectory Towards Alpha Apex Target/4(phi) -> Mux8/1
  Virtual Leg Trajectory Towards Alpha Apex Target/5(dphi) -> Mux8/2
  Virtual Leg Trajectory Towards Alpha Apex Target/6(ddphi) -> Mux8/3
  Mux6/1 -> Mux7/2
  Mux5/1 -> Mux7/1
  Selector/1 -> Virtual Leg Trajectory Towards Alpha Apex Target/3(theta)
  Torso Pitch [rad rad/s]/1 -> Selector/1
  Mux10/1 -> Switch/1
  Mux8/1 -> Mux10/2
  Mux9/1 -> Mux10/1
  Switch/1 -> Demux6/1
  Mux7/1 -> Switch/3
  Move Leg to Apex Target [1/0]/1 -> Switch/2, Detect Change/1
  Fcn2/1 -> Mux6/1
  k_virtual6/1 -> Mux6/2
  Constant4/1 -> Mux6/3
  Constant1/1 -> Mux5/1
  Constant3/1 -> Mux5/3
  Constant2/1 -> Mux5/2
  Gain5/1 -> Demux5/1
  Primary Front Gear [rad rad/s]/1 -> Sum4/2
  Primary Back Gear [rad rad/s]/1 -> Sum4/1
  Sum4/1 -> Gain5/1
  Demux5/1 -> Fcn2/1
  Demux5/2 -> k_virtual6/1
  Back/Front Motor PD/1(Commanded Torque [Nm] [back front]) -> Secondary Back/Front Motor Torque [Nm Nm]/1
  Constant5/1 -> Secondary Force or Position Control [1/0]/1

== system spring_mass_model_01/Control/Behavior Control/Torque Distribution Left ==
  Leg Torque [Nm] : Inport
  Leg Force [N] : Inport  Port=2
  w [m] : Inport  Port=3
  Gain : Gain  Gain=0.5
  Gain1 : Gain  Gain=0.5
  Motor Torque Saturation Optimization : MATLAB Function  TreatAsAtomicUnit=on
  Product : Product  RndMeth=Zero
  Sum : Sum  Inputs=|++
  Sum1 : Sum  Inputs=+-|
  Back Torque [Nm] : Outport
  Front Torque [Nm] : Outport  Port=2
  wires:
  Sum1/1 -> Back Torque [Nm]/1
  Leg Torque [Nm]/1 -> Gain/1
  Sum/1 -> Front Torque [Nm]/1
  Motor Torque Saturation Optimization/1(t1) -> Sum/1, Sum1/1
  w [m]/1 -> Product/2
  Motor Torque Saturation Optimization/2(t2) -> Sum1/2, Sum/2
  Leg Force [N]/1 -> Product/1
  Product/1 -> Gain1/1
  Gain1/1 -> Motor Torque Saturation Optimization/2(x2s)
  Gain/1 -> Motor Torque Saturation Optimization/1(x1s)

== system spring_mass_model_01/Control/Behavior Control/Torque Distribution Right ==
  Leg Torque [Nm] : Inport
  Leg Force [N] : Inport  Port=2
  w [m] : Inport  Port=3
  Gain : Gain  Gain=0.5
  Gain1 : Gain  Gain=0.5
  Motor Torque Saturation Optimization : MATLAB Function  TreatAsAtomicUnit=on
  Product : Product  RndMeth=Zero
  Sum : Sum  Inputs=|++
  Sum1 : Sum  Inputs=+-|
  Back Torque [Nm] : Outport
  Front Torque [Nm] : Outport  Port=2
  wires:
  Gain/1 -> Motor Torque Saturation Optimization/1(x1s)
  Gain1/1 -> Motor Torque Saturation Optimization/2(x2s)
  Product/1 -> Gain1/1
  Leg Force [N]/1 -> Product/1
  Motor Torque Saturation Optimization/2(t2) -> Sum/2, Sum1/2
  w [m]/1 -> Product/2
  Motor Torque Saturation Optimization/1(t1) -> Sum1/1, Sum/1
  Sum/1 -> Front Torque [Nm]/1
  Leg Torque [Nm]/1 -> Gain/1
  Sum1/1 -> Back Torque [Nm]/1

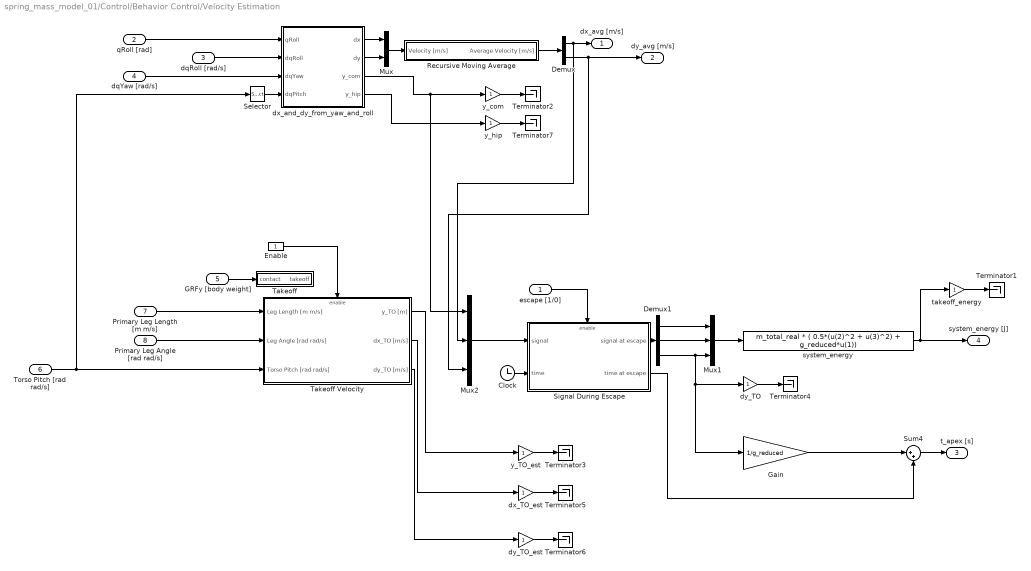
== system spring_mass_model_01/Control/Behavior Control/Velocity Estimation ==
  escape [1/0] : Inport
  qRoll [rad] : Inport  Port=2
  dqRoll [rad/s] : Inport  Port=3
  dqYaw [rad/s] : Inport  Port=4
  GRFy [body weight] : Inport  Port=5
  Torso Pitch [rad rad/s] : Inport  Port=6
  Primary Leg Length [m m/s] : Inport  Port=7
  Primary Leg Angle [rad rad/s] : Inport  Port=8
  Clock : Clock
  Demux : Demux  Outputs=2
  Demux1 : Demux  Outputs=3
  Enable : Constant  OutDataTypeStr=boolean
  Gain : Gain  Gain=1/g_reduced
  Mux : Mux  Inputs=2
  Mux1 : Mux  Inputs=3
  Mux2 : Mux  Inputs=3
  Recursive Moving Average : Subsystem
  Selector : Selector  InputPortWidth=2  Indices=[2]
  Signal During Escape : Subsystem
  Sum4 : Sum  Inputs=|++
  Takeoff : Subsystem
  Takeoff Velocity : Subsystem
  Terminator{1..7} (7 alike) : Terminator
  dx_TO_est : Gain
  dx_and_dy_from_yaw_and_roll : MATLAB Function  TreatAsAtomicUnit=on
  dy_TO : Gain
  dy_TO_est : Gain
  system_energy : Fcn  Expr=m_total_real * ( 0.5*(u(2)^2 + u(3)^2) + g_reduced*u(1))
  takeoff_energy : Gain
  y_TO_est : Gain
  y_com : Gain
  y_hip : Gain
  dx_avg [m/s] : Outport
  dy_avg [m/s] : Outport  Port=2
  t_apex [s] : Outport  Port=3
  system_energy [J] : Outport  Port=4
  wires:
  Recursive Moving Average/1(Average Velocity [m/s]) -> Demux/1
  dx_and_dy_from_yaw_and_roll/1(dx) -> Mux/1
  dqYaw [rad/s]/1 -> dx_and_dy_from_yaw_and_roll/3(dqYaw)
  Selector/1 -> dx_and_dy_from_yaw_and_roll/4(dqPitch)
  GRFy [body weight]/1 -> Takeoff/1(contact)
  dx_and_dy_from_yaw_and_roll/2(dy) -> Mux/2
  Mux/1 -> Recursive Moving Average/1(Velocity [m/s])
  Demux/1 -> Mux2/2, dx_avg [m/s]/1
  Demux/2 -> Mux2/3, dy_avg [m/s]/1
  Sum4/1 -> t_apex [s]/1
  Primary Leg Length [m m/s]/1 -> Takeoff Velocity/1(Leg Length [m m/s])
  Primary Leg Angle [rad rad/s]/1 -> Takeoff Velocity/2(Leg Angle [rad rad/s])
  Torso Pitch [rad rad/s]/1 -> Selector/1, Takeoff Velocity/3(Torso Pitch [rad rad/s])
  Demux1/2 -> Mux1/2
  Demux1/1 -> Mux1/1
  Mux1/1 -> system_energy/1
  dy_TO/1 -> Terminator4/1
  takeoff_energy/1 -> Terminator1/1
  dqRoll [rad/s]/1 -> dx_and_dy_from_yaw_and_roll/2(dqRoll)
  escape [1/0]/1 -> Signal During Escape/Enable
  Mux2/1 -> Signal During Escape/1(signal)
  Signal During Escape/1(signal at escape) -> Demux1/1
  qRoll [rad]/1 -> dx_and_dy_from_yaw_and_roll/1(qRoll)
  dx_and_dy_from_yaw_and_roll/3(y_com) -> Mux2/1, y_com/1
  Signal During Escape/2(time at escape) -> Sum4/2
  Demux1/3 -> Gain/1, dy_TO/1, Mux1/3
  Clock/1 -> Signal During Escape/2(time)
  system_energy/1 -> system_energy [J]/1, takeoff_energy/1
  y_com/1 -> Terminator2/1
  Takeoff Velocity/1(y_TO [m]) -> y_TO_est/1
  y_TO_est/1 -> Terminator3/1
  dx_TO_est/1 -> Terminator5/1
  Takeoff Velocity/2(dx_TO [m/s]) -> dx_TO_est/1
  dy_TO_est/1 -> Terminator6/1
  Takeoff Velocity/3(dy_TO [m/s]) -> dy_TO_est/1
  y_hip/1 -> Terminator7/1
  dx_and_dy_from_yaw_and_roll/4(y_hip) -> y_hip/1
  Enable/1 -> Takeoff Velocity/Enable
  Gain/1 -> Sum4/1

== system spring_mass_model_01/Control/Behavior Control/Virtual Spring Calculator ==
  "Stance Leg Angle [rad rad/s] " : Inport
  Stance Leg Length [m m/s] : Inport  Port=2
  Torso Angle [rad rad/s] : Inport  Port=3
  Demux : Demux  Outputs=2
  Demux1 : Demux  Outputs=2
  Demux2 : Demux  Outputs=2
  Mux3 : Mux  Inputs=2
  Mux4 : Mux  Inputs=2
  Virtual Spring Calculations : MATLAB Function  TreatAsAtomicUnit=on
  Spring Length [m m/s] : Outport
  Spring Alpha [rad rad/s] : Outport  Port=2  OutDataTypeStr=double  PortDimensions=2
  wires:
  Mux4/1 -> Spring Alpha [rad rad/s]/1
  Virtual Spring Calculations/4(dl_v) -> Mux3/2
  Virtual Spring Calculations/3(l_v) -> Mux3/1
  Virtual Spring Calculations/2(dalpha_v) -> Mux4/2
  Virtual Spring Calculations/1(alpha_v) -> Mux4/1
  Demux1/2 -> Virtual Spring Calculations/4(dl)
  Demux2/2 -> Virtual Spring Calculations/6(dphi)
  Demux2/1 -> Virtual Spring Calculations/5(phi)
  Demux1/1 -> Virtual Spring Calculations/3(l)
  Demux/2 -> Virtual Spring Calculations/2(dth)
  Demux/1 -> Virtual Spring Calculations/1(th)
  Torso Angle [rad rad/s]/1 -> Demux/1
  "Stance Leg Angle [rad rad/s] "/1 -> Demux2/1
  Mux3/1 -> Spring Length [m m/s]/1
  Stance Leg Length [m m/s]/1 -> Demux1/1
